simulink model "verify_Controller_Bang_Bang_mdl"  (R2016b)
settings: Solver=VariableStepDiscrete  StartTime=0.0  StopTime=2.5  MaxStep=0.1  RelTol=1e-3  EnableMultiTasking=on
libraries: carnot x1, simulink x1
settings Model: Creator=drhf  LastModifiedBy=srrt
settings DataIOCC: SaveFormat=Array  SignalLoggingSaveFormat=ModelDataLogs
settings OptimizationCC: ExpressionDepthLimit=2147483647  LifeSpan=inf
settings DebuggingCC: UnderspecifiedInitializationDetection=Classic  MergeDetectMultiDrivingBlocksExec=none  SolverPrmCheckMsg=warning  FcnCallInpInsideContextMsg=warning  StateNameClashWarn=warning  SFUnexpectedBacktrackingDiag=warning  SFNoUnconditionalDefaultTransitionDiag=warning  SFExecutionAtInitializationDiag=none
settings HardwareCC: ProdBitPerPointer=32  ProdBitPerSizeT=32  ProdBitPerPtrDiffT=32  ProdLargestAtomicFloat=None  ProdIntDivRoundTo=Undefined  ProdEndianess=Unspecified  ProdWordSize=32  ProdHWDeviceType=32-bit Generic
settings ModelReferenceCC: PropagateSignalLabelsOutOfModel=off
settings GRTTargetCC: TargetLangStandard=C89/C90 (ANSI)  GeneratePreprocessorConditionals=Disable all  CombineOutputUpdateFcns=off  GRTInterface=on
settings ConfigComp: CovMetricSettings=dw  CovHtmlReporting=on  CovSaveCumulativeToWorkspaceVar=on  CovSaveSingleToWorkspaceVar=on  CovExternalEMLEnable=off

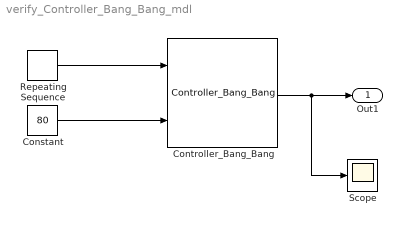
== system verify_Controller_Bang_Bang_mdl ==
  Constant : Constant  Value=80
  Controller_Bang_Bang : carnot/Control/Controller_Bang_Bang  deltaTon=5  deltaToff=1  Tmax=90
  Repeating Sequence : simulink/Sources/Repeating Sequence  rep_seq_t=[0 0.5 0.6 1 1.1 1.5 1.6 2 2.1 2.5]  rep_seq_y=[80 80 85 85 91 91 86 86 81 81]
  Scope : Scope
  Out1 : Outport
  wires:
  Controller_Bang_Bang/1 -> Scope/1, Out1/1
  Constant/1 -> Controller_Bang_Bang/2
  Repeating Sequence/1 -> Controller_Bang_Bang/1
